simulink model "Model"  (R2021b)
settings: Solver=FixedStepAuto  StartTime=0.0  StopTime=T  FixedStep=0.1  RelTol=1e-3
values from neighbouring files (symbols this model uses):
  a = R_E + 550    [Model_script_291.m]
  A0 = eye(3)    [Model_script_291.m]
  actuators_matrix = [1 0 0; 0 1 0; 0 0 1]    [Model_script_291.m]
  alpha = deg2rad(11.5)    [Model_script_291.m]
  Area_mb = diag([A1 A2 A3 A4 A5 A6])    [Model_script_291.m]
  Area_sp = diag([A7 A8 A9 A10])    [Model_script_291.m]
  around_boresight = deg2rad(dms2degrees([0,0,around_boresight]))    [Model_script_291.m]
  cross_boresight = deg2rad(dms2degrees([0,0,cross_boresight]))    [Model_script_291.m]
  e = 0.0001824    [Model_script_291.m]
  epsilon = deg2rad(23.45)    [Model_script_291.m]
  H0 = ( g1_0^2 + g1_1^2 + h1_1^2 )^(1/2)    (= 3.0115258674e-05)    [Model_script_291.m]
  I = I_mb + I_depl    [Model_script_291.m]
  i = deg2rad(53.0545)    [Model_script_291.m]
  I_inv = inv(I)    [Model_script_291.m]
  i_matrix = [1 0 0; 0 cos(i) sin(i); 0 -sin(i) cos(i)]    [Model_script_291.m]
  Kb = 1e10    (= 10000000000)    [Model_script_291.m]
  Kd_slew = [5e-5; 5e-5; 5e-5]    [Model_script_291.m]
  Kd_tracking = [5e-3; 0.8*(5e-3); 5e-3]    [Model_script_291.m]
  Kp_slew = [5e-4; 5e-4; 5e-4]    [Model_script_291.m]
  Kp_tracking = [5e-2; 5e-2; 5e-2]    [Model_script_291.m]
  m = [0.01; 0.05; 0.01]    [Model_script_291.m]
  m_N_unit = zeros(size(m_N,1),size(m_N,2))    [Model_script_291.m]
  mu_E = astroConstants(13)    [Model_script_291.m]
  n = sqrt(mu_E/(a^3))    [Model_script_291.m]
  n4 = -n1    [Model_script_291.m]
  N_b_mb = [n1'; n2'; n3'; n4'; n5'; n6']    [Model_script_291.m]
  N_b_sp = [n7'; n8'; n9'; n10']    [Model_script_291.m]
  n_sun = 2*pi/T_sun    (= 1.99238499086e-07)    [Model_script_291.m]
  P = Fe/c    (= 4.52666666667e-06)    [Model_script_291.m]
  R_E = astroConstants(23)    [Model_script_291.m]
  r_mb = [base/2 0 0; 0 base/2 0; 0 0 height/2; -base/2 0 0; 0 -base/2 0; 0 0 -height/2]    [Model_script_291.m]
  r_sp = [0 length_p1/2+base/2 0; 0 length_p1/2+base/2 0; 0 -length_p2/2-base/2 0; 0 -length_p2/2-base/2 0]    [Model_script_291.m]
  rho_s_mb = 0.3    [Model_script_291.m]
  rho_s_sp = 0    [Model_script_291.m]
  Rs = astroConstants(2)    [Model_script_291.m]
  star_sensor_tolerance = deg2rad(star_sensor_tolerance)    [Model_script_291.m]
  theta0 = deg2rad(0)    [Model_script_291.m]
  unit = [1 0 0]'    [Model_script_291.m]
  v1 = [0 1 -1]'    [Model_script_291.m]
  v2 = [-1 0 1]'    [Model_script_291.m]
  v3 = [1 -1 0]'    [Model_script_291.m]
  w_0 = [wx_0 wy_0 wz_0]'    [Model_script_291.m]
  w_E = deg2rad(15.04)/3600    [Model_script_291.m]
  w_target = [0; 0; n]    [Model_script_291.m]
  weight = 1/6    (= 0.166666666667)    [Model_script_291.m]
  wy_0 = 0.7    [Model_script_291.m]
libraries: matrix_library x16, vrlib x12, dspmtrx3 x2, sharedutil x2
(part 1 of 2)
settings Model: Creator=sferl  LastModifiedBy=samuz

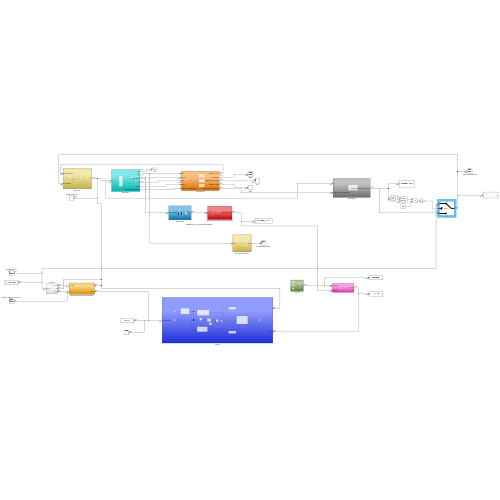
[thumbnail: Simulink's stored preview of the top-level diagram]
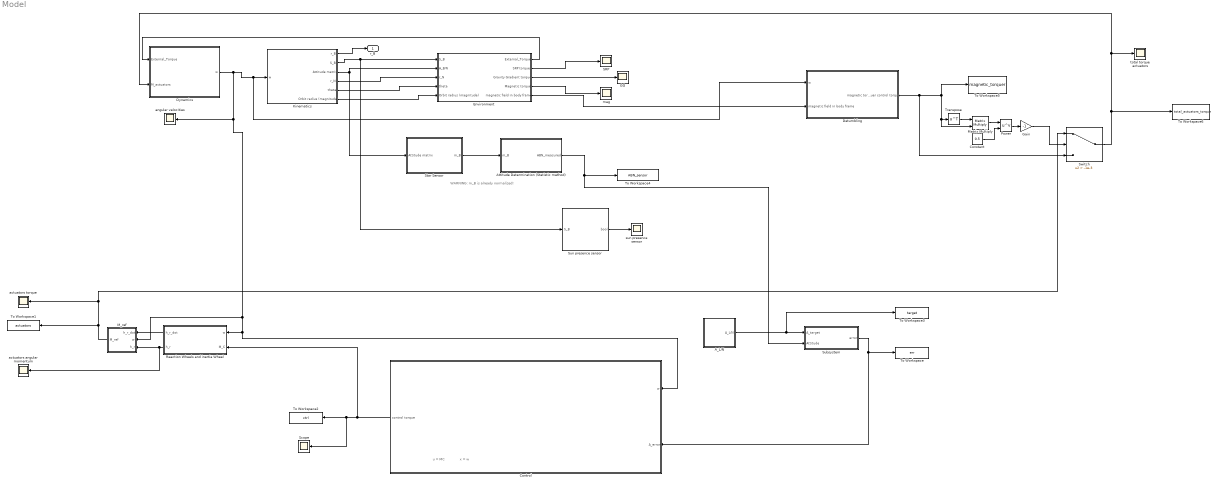
== system Model ==
  note: x = w
  note: u = MC
  note: WARNING: m_B is already normalized!
  A_L/N : Subsystem
  Attitude Determination (Statistic method) : Subsystem
  Constant : Constant  Value=0.5
  Control : Subsystem
  Detumbling : Subsystem
  Dynamics : Subsystem
  Environment : Subsystem
  GG : Scope
  Gain : Gain  Gain=-1
  Kinematics : Subsystem
  M_ref : Subsystem
  Matrix Multiply : Product  Multiplication=Matrix(*)
  Power : Math  Operator=pow  SaturateOnIntegerOverflow=on
  Reaction Wheels and inertia Wheel : Subsystem
  SRP : Scope
  Scope : Scope
  Star Sensor : Subsystem
  Subsystem : Subsystem
  Sun presence sensor : Subsystem
  Switch : Switch  Criteria=u2 > Threshold  Threshold=-1e-3
  To Workspace : ToWorkspace  VariableName=err  SampleTime=-1
  To Workspace1 : ToWorkspace  VariableName=actuators  SampleTime=-1
  To Workspace2 : ToWorkspace  VariableName=ctrl  SampleTime=-1
  To Workspace3 : ToWorkspace  VariableName=target  SampleTime=-1
  To Workspace4 : ToWorkspace  VariableName=ABN_sensor  SampleTime=-1
  To Workspace5 : ToWorkspace  VariableName=magnetic_torquer  SampleTime=-1
  To Workspace6 : ToWorkspace  VariableName=total_actuators_torque  SampleTime=-1
  Transpose : Math  Operator=transpose  SaturateOnIntegerOverflow=on
  actuators angular momentum : Scope
  actuators torque : Scope
  angular velocities : Scope
  mag : Scope
  sun presence sensor : Scope
  total torque actuators : Scope
  r_B : Outport
  wires:
  Kinematics/1(r_B) -> r_B/1
  Kinematics/3(Attitude matrix) -> Environment/2(A_B/N), Star Sensor/1(Attitude matrix)
  Star Sensor/1(m_B) -> Attitude Determination (Statistic method)/1(m_B)
  Kinematics/2(S_B) -> Sun presence sensor/1(S_B), Environment/1(S_B)
  Kinematics/4(r_N) -> Environment/3(r_N)
  Kinematics/5(theta) -> Environment/4(theta)
  Kinematics/6(Orbit radius (magnitude)) -> Environment/5(Orbit radius (magnitude))
  Environment/1(External_Torque) -> Dynamics/1(External_Torque)
  Attitude Determination (Statistic method)/1(ABN_measured) -> To Workspace4/1, Subsystem/2(Attitude)
  Subsystem/1(error) -> Control/2(A_error), To Workspace/1
  Environment/2(SRP torque) -> SRP/1
  Environment/3(Gravity Gradient torque) -> GG/1
  Environment/4(Magnetic torque) -> mag/1
  A_L/N/1(A_L/N) -> To Workspace3/1, Subsystem/1(A_target)
  Environment/5(magnetic field in body frame) -> Detumbling/2(magnetic field in body frame)
  Detumbling/1(magnetic torquer control torque) -> Switch/3, To Workspace5/1, Matrix Multiply/2, Transpose/1
  Dynamics/1(w) -> Detumbling/1(w), Kinematics/1(w), M_ref/2(w), Reaction Wheels and inertia Wheel/1(w), Control/1(w), angular velocities/1
  Transpose/1 -> Matrix Multiply/1
  Constant/1 -> Power/2
  Matrix Multiply/1 -> Power/1
  Power/1 -> Gain/1
  Gain/1 -> Switch/2
  Reaction Wheels and inertia Wheel/1(h_r_dot) -> M_ref/1(h_r_dot)
  Reaction Wheels and inertia Wheel/2(h_r) -> M_ref/3(h_r), actuators angular momentum/1
  Control/1(control torque) -> Reaction Wheels and inertia Wheel/2(M_C), Scope/1, To Workspace2/1
  M_ref/1(M_ref) -> To Workspace1/1, Switch/1, actuators torque/1
  Sun presence sensor/1(bool) -> sun presence sensor/1
  Switch/1 -> Dynamics/2(M_actuators), total torque actuators/1, To Workspace6/1

== system Model/A_L//N ==
  Matrix Concatenate : Concatenate  NumInputs=3  Mode=Multidimensional array  ConcatenateDimension=2
  first column of A_L/N : Subsystem
  second column of A_L/N : Subsystem
  third column of A_L/N : Subsystem
  A_L/N : Outport
  wires:
  second column of A_L/N/1(A_L/N (:,2)) -> Matrix Concatenate/2
  Matrix Concatenate/1 -> A_L/N/1
  first column of A_L/N/1(A_L/N (:,1)) -> Matrix Concatenate/1
  third column of A_L/N/1(A_L/N (:,3)) -> Matrix Concatenate/3

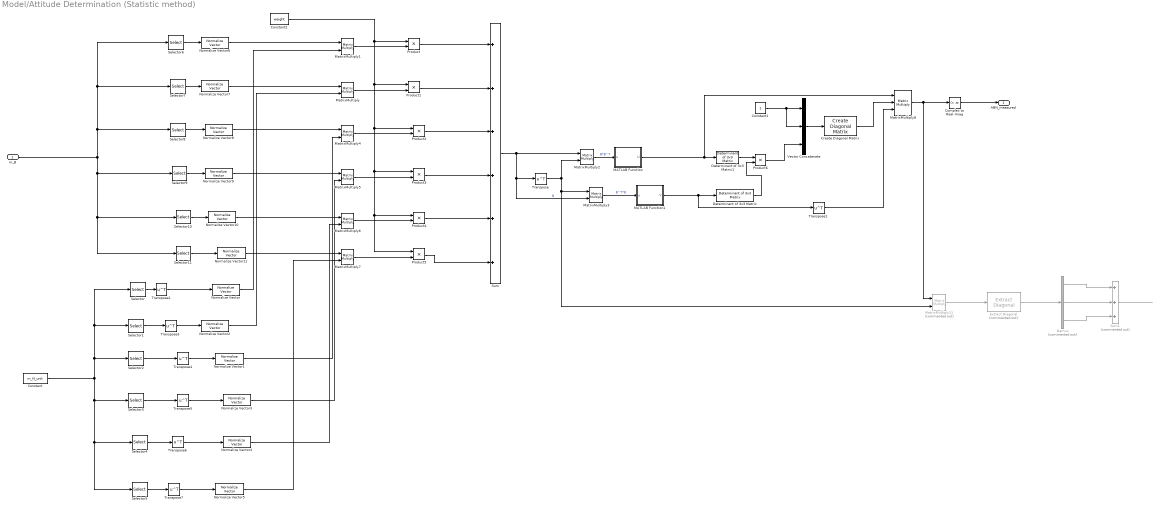
== system Model/Attitude Determination (Statistic method) ==
  m_B : Inport
  Complex to Real-Imag : ComplexToRealImag  Output=Real
  Constant : Constant  Value=m_N_unit
  Constant1 : Constant
  Constant2 : Constant  Value=weight
  Create Diagonal Matrix : dspmtrx3/Create Diagonal Matrix
      settings: SourceProductBaseCode=DS
  Demux : Demux  Commented=on  Outputs=3
  Determinant of 3x3 Matrix : sharedutil/Determinant of 3x3 Matrix  aMode=aMode
      settings: SourceProductBaseCode=AE,PW,DR,MT,UV,VE
  Determinant of 3x3 Matrix1 : sharedutil/Determinant of 3x3 Matrix  aMode=aMode
      settings: SourceProductBaseCode=AE,PW,DR,MT,UV,VE
  Extract Diagonal : dspmtrx3/Extract Diagonal  Commented=on
      settings: SourceProductBaseCode=DS
  MATLAB Function : MATLAB Function  TreatAsAtomicUnit=on
  MATLAB Function1 : MATLAB Function  TreatAsAtomicUnit=on
  MatrixMultiply{,1..7} (8 alike) : Product  Multiplication=Matrix(*)
  MatrixMultiply11 : Product  Commented=on  Multiplication=Matrix(*)
  MatrixMultiply8 : Product  Inputs=3  Multiplication=Matrix(*)
  Normalize Vector{,1..11} (12 alike) : vrlib/Utilities/Normalize Vector  maxzero=0
  Product{,1..6} (7 alike) : Product
  Selector : Selector  NumberOfDimensions=2  InputPortWidth=3  IndexOptions=Starting index (dialog),Starting index (dialog)  Indices=1,1  OutputSizes=3,1
  Selector1 : Selector  NumberOfDimensions=2  InputPortWidth=3  IndexOptions=Starting index (dialog),Starting index (dialog)  Indices=1,2  OutputSizes=3,1
  Selector10 : Selector  NumberOfDimensions=2  InputPortWidth=3  IndexOptions=Starting index (dialog),Starting index (dialog)  Indices=1,5  OutputSizes=3,1
  Selector11 : Selector  NumberOfDimensions=2  InputPortWidth=3  IndexOptions=Starting index (dialog),Starting index (dialog)  Indices=1,6  OutputSizes=3,1
  Selector2 : Selector  NumberOfDimensions=2  InputPortWidth=3  IndexOptions=Starting index (dialog),Starting index (dialog)  Indices=1,3  OutputSizes=3,1
  Selector3 : Selector  NumberOfDimensions=2  InputPortWidth=3  IndexOptions=Starting index (dialog),Starting index (dialog)  Indices=1,4  OutputSizes=3,1
  Selector4 : Selector  NumberOfDimensions=2  InputPortWidth=3  IndexOptions=Starting index (dialog),Starting index (dialog)  Indices=1,5  OutputSizes=3,1
  Selector5 : Selector  NumberOfDimensions=2  InputPortWidth=3  IndexOptions=Starting index (dialog),Starting index (dialog)  Indices=1,6  OutputSizes=3,1
  Selector6 : Selector  NumberOfDimensions=2  InputPortWidth=3  IndexOptions=Starting index (dialog),Starting index (dialog)  Indices=1,1  OutputSizes=3,1
  Selector7 : Selector  NumberOfDimensions=2  InputPortWidth=3  IndexOptions=Starting index (dialog),Starting index (dialog)  Indices=1,2  OutputSizes=3,1
  Selector8 : Selector  NumberOfDimensions=2  InputPortWidth=3  IndexOptions=Starting index (dialog),Starting index (dialog)  Indices=1,3  OutputSizes=3,1
  Selector9 : Selector  NumberOfDimensions=2  InputPortWidth=3  IndexOptions=Starting index (dialog),Starting index (dialog)  Indices=1,4  OutputSizes=3,1
  Sum : Sum  Inputs=++++++
  Sum1 : Sum  Commented=on  Inputs=+++
  Transpose{,1..7} (8 alike) : Math  Operator=transpose  SaturateOnIntegerOverflow=on
  Vector Concatenate : Concatenate  NumInputs=3
  ABN_measured : Outport
  wires:
  Transpose/1 -> MatrixMultiply11/2, MatrixMultiply3/1, MatrixMultiply2/2
  Constant2/1 -> Product3/1, Product4/1, Product5/1, Product2/1, Product1/1, Product/1
  Product2/1 -> Sum/3
  MatrixMultiply/1 -> Product1/2
  Product1/1 -> Sum/2
  MatrixMultiply7/1 -> Product5/2
  Sum/1 -> MatrixMultiply3/2, Transpose/1, MatrixMultiply2/1  "B"
  MatrixMultiply2/1 -> MATLAB Function/1(u)  "B*B^T"
  Product5/1 -> Sum/6
  MatrixMultiply5/1 -> Product3/2
  Product4/1 -> Sum/5
  Product/1 -> Sum/1
  MatrixMultiply4/1 -> Product2/2
  MatrixMultiply1/1 -> Product/2
  Product3/1 -> Sum/4
  MatrixMultiply6/1 -> Product4/2
  Selector1/1 -> Transpose3/1
  Selector3/1 -> Transpose5/1
  Selector4/1 -> Transpose6/1
  Selector2/1 -> Transpose4/1
  Selector5/1 -> Transpose7/1
  m_B/1 -> Selector6/1, Selector7/1, Selector8/1, Selector11/1, Selector10/1, Selector9/1
  Determinant of 3x3 Matrix1/1 -> Product6/1
  Determinant of 3x3 Matrix/1 -> Product6/2
  Constant1/1 -> Vector Concatenate/2, Vector Concatenate/1
  Product6/1 -> Vector Concatenate/3
  Vector Concatenate/1 -> Create Diagonal Matrix/1
  Create Diagonal Matrix/1 -> MatrixMultiply8/2
  MATLAB Function/1(U) -> MatrixMultiply8/1, Determinant of 3x3 Matrix1/1
  Transpose1/1 -> MatrixMultiply8/3
  MatrixMultiply8/1 -> Complex to Real-Imag/1, MatrixMultiply11/1
  MatrixMultiply3/1 -> MATLAB Function1/1(u)  "B^T*B"
  MATLAB Function1/1(V) -> Transpose1/1, Determinant of 3x3 Matrix/1
  MatrixMultiply11/1 -> Extract Diagonal/1
  Extract Diagonal/1 -> Demux/1
  Demux/1 -> Sum1/1
  Demux/2 -> Sum1/2
  Demux/3 -> Sum1/3
  Sum1/1 -> ?
  Selector6/1 -> Normalize Vector6/1
  Selector7/1 -> Normalize Vector7/1
  Selector8/1 -> Normalize Vector8/1
  Selector9/1 -> Normalize Vector9/1
  Selector10/1 -> Normalize Vector10/1
  Selector11/1 -> Normalize Vector11/1
  Selector/1 -> Transpose2/1
  Transpose3/1 -> Normalize Vector2/1
  Transpose2/1 -> Normalize Vector/1
  Transpose4/1 -> Normalize Vector1/1
  Transpose5/1 -> Normalize Vector3/1
  Transpose6/1 -> Normalize Vector4/1
  Transpose7/1 -> Normalize Vector5/1
  Normalize Vector/1 -> MatrixMultiply1/2
  Normalize Vector2/1 -> MatrixMultiply/2
  Normalize Vector1/1 -> MatrixMultiply4/2
  Normalize Vector3/1 -> MatrixMultiply5/2
  Normalize Vector4/1 -> MatrixMultiply6/2
  Normalize Vector5/1 -> MatrixMultiply7/2
  Normalize Vector6/1 -> MatrixMultiply1/1
  Normalize Vector7/1 -> MatrixMultiply/1
  Normalize Vector8/1 -> MatrixMultiply4/1
  Normalize Vector9/1 -> MatrixMultiply5/1
  Normalize Vector10/1 -> MatrixMultiply6/1
  Normalize Vector11/1 -> MatrixMultiply7/1
  Constant/1 -> Selector3/1, Selector4/1, Selector5/1, Selector/1, Selector1/1, Selector2/1
  Complex to Real-Imag/1 -> ABN_measured/1

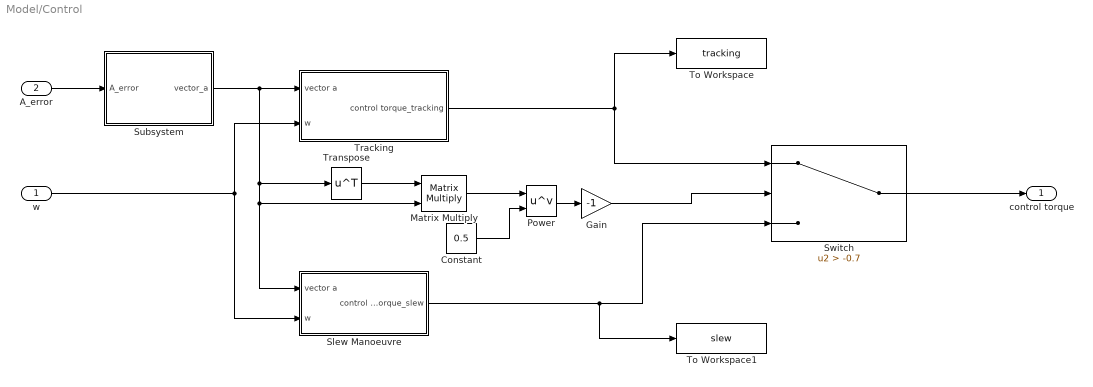
== system Model/Control ==
  w : Inport
  A_error : Inport  Port=2
  Constant : Constant  Value=0.5
  Gain : Gain  Gain=-1
  Matrix Multiply : Product  Multiplication=Matrix(*)
  Power : Math  Operator=pow  SaturateOnIntegerOverflow=on
  Slew Manoeuvre : Subsystem
  Subsystem : Subsystem
  Switch : Switch  Criteria=u2 > Threshold  Threshold=-0.7
  To Workspace : ToWorkspace  VariableName=tracking  SampleTime=-1
  To Workspace1 : ToWorkspace  VariableName=slew  SampleTime=-1
  Tracking : Subsystem
  Transpose : Math  Operator=transpose  SaturateOnIntegerOverflow=on
  control torque : Outport
  wires:
  w/1 -> Tracking/2(w), Slew Manoeuvre/2(w)
  Tracking/1(control torque_tracking) -> Switch/1, To Workspace/1
  A_error/1 -> Subsystem/1(A_error)
  Subsystem/1(vector_a) -> Slew Manoeuvre/1(vector a), Matrix Multiply/2, Transpose/1, Tracking/1(vector a)
  Slew Manoeuvre/1(control torque_slew) -> Switch/3, To Workspace1/1
  Switch/1 -> control torque/1
  Transpose/1 -> Matrix Multiply/1
  Matrix Multiply/1 -> Power/1
  Gain/1 -> Switch/2
  Constant/1 -> Power/2
  Power/1 -> Gain/1

== system Model/Detumbling ==
  w : Inport
  magnetic field in body frame : Inport  Port=2
  Mangetic Torquer : Subsystem
  magnetic torquer control torque : Outport
  wires:
  w/1 -> Mangetic Torquer/1(w)
  magnetic field in body frame/1 -> Mangetic Torquer/2(b)
  Mangetic Torquer/1(M_C) -> magnetic torquer control torque/1

== system Model/Dynamics ==
  External_Torque : Inport
  M_actuators : Inport  Port=2
  Constant : Constant  Value=I  VectorParams1D=off
  Constant1 : Constant  Value=I_inv  VectorParams1D=off
  Cross Product : matrix_library/Cross Product
      settings: SourceProductBaseCode=SL
  Integrator : Integrator  InitialCondition=w_0
  Product : Product  Multiplication=Matrix(*)
  Product1 : Product  Multiplication=Matrix(*)
  Sum : Sum  Inputs=|++
  Sum1 : Sum  Inputs=|++
  w : Outport
  wires:
  Product/1 -> Cross Product/1
  Constant/1 -> Product/1
  Constant1/1 -> Product1/1
  Integrator/1 -> Cross Product/2, Product/2, w/1  "w"
  Product1/1 -> Integrator/1  "w_dot"
  Cross Product/1 -> Sum/2
  Sum/1 -> Product1/2
  External_Torque/1 -> Sum1/1
  M_actuators/1 -> Sum1/2
  Sum1/1 -> Sum/1

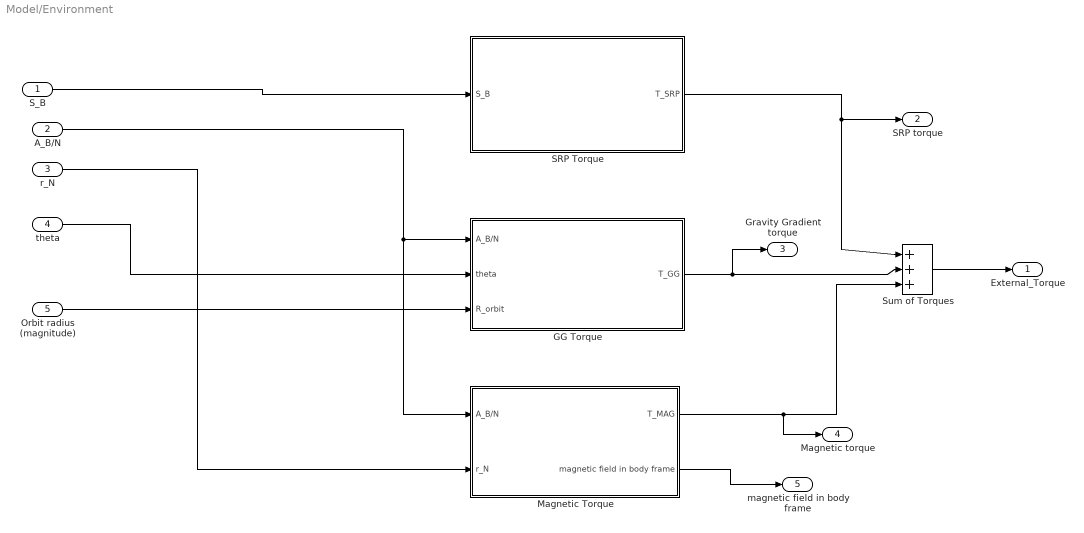
== system Model/Environment ==
  S_B : Inport
  A_B/N : Inport  Port=2
  r_N : Inport  Port=3
  theta : Inport  Port=4
  Orbit radius (magnitude) : Inport  Port=5
  GG Torque : Subsystem
  Magnetic Torque : Subsystem
  SRP Torque : Subsystem
  Sum of Torques : Sum  Inputs=+|+|+  CollapseMode=Specified dimension
  External_Torque : Outport
  SRP torque : Outport  Port=2
  Gravity Gradient torque : Outport  Port=3
  Magnetic torque : Outport  Port=4
  magnetic field in body frame : Outport  Port=5
  wires:
  SRP Torque/1(T_SRP) -> SRP torque/1, Sum of Torques/1
  r_N/1 -> Magnetic Torque/2(r_N)
  GG Torque/1(T_GG) -> Gravity Gradient torque/1, Sum of Torques/2
  A_B/N/1 -> Magnetic Torque/1(A_B/N), GG Torque/1(A_B/N)
  Orbit radius (magnitude)/1 -> GG Torque/3(R_orbit)
  Magnetic Torque/1(T_MAG) -> Magnetic torque/1, Sum of Torques/3
  Sum of Torques/1 -> External_Torque/1
  S_B/1 -> SRP Torque/1(S_B)
  theta/1 -> GG Torque/2(theta)
  Magnetic Torque/2(magnetic field in body frame) -> magnetic field in body frame/1

== system Model/Kinematics ==
  w : Inport
  Sun direction with respect to body frame (already normalized!) : Subsystem
  "radius of orbit in body frame and transformation matrix from inertial frame to body frame " : Subsystem
  r_B : Outport
  S_B : Outport  Port=2
  Attitude matrix : Outport  Port=3
  r_N : Outport  Port=4
  theta : Outport  Port=5
  Orbit radius (magnitude) : Outport  Port=6
  wires:
  "radius of orbit in body frame and transformation matrix from inertial frame to body frame "/1(r_B) -> r_B/1
  w/1 -> "radius of orbit in body frame and transformation matrix from inertial frame to body frame "/1(w)
  Sun direction with respect to body frame (already normalized!)/1(S_B) -> S_B/1
  "radius of orbit in body frame and transformation matrix from inertial frame to body frame "/3(r_N) -> r_N/1
  "radius of orbit in body frame and transformation matrix from inertial frame to body frame "/4(theta) -> theta/1
  "radius of orbit in body frame and transformation matrix from inertial frame to body frame "/5(R_orbit) -> Orbit radius (magnitude)/1
  "radius of orbit in body frame and transformation matrix from inertial frame to body frame "/2(A_B/N) -> Attitude matrix/1, Sun direction with respect to body frame (already normalized!)/1(A_B/N)

== system Model/M_ref ==
  h_r_dot : Inport
  w : Inport  Port=2
  h_r : Inport  Port=3
  Constant : Constant  Value=actuators_matrix
  Constant1 : Constant  Value=actuators_matrix
  Cross Product : matrix_library/Cross Product
      settings: SourceProductBaseCode=SL
  Gain : Gain  Gain=-1
  MatrixMultiply : Product  Multiplication=Matrix(*)
  MatrixMultiply1 : Product  Multiplication=Matrix(*)
  Sum : Sum  Inputs=|++
  M_ref : Outport
  wires:
  MatrixMultiply1/1 -> Cross Product/2
  MatrixMultiply/1 -> Sum/1
  Sum/1 -> Gain/1
  Constant/1 -> MatrixMultiply/1
  h_r_dot/1 -> MatrixMultiply/2
  Cross Product/1 -> Sum/2
  Gain/1 -> M_ref/1
  w/1 -> Cross Product/1
  Constant1/1 -> MatrixMultiply1/1
  h_r/1 -> MatrixMultiply1/2

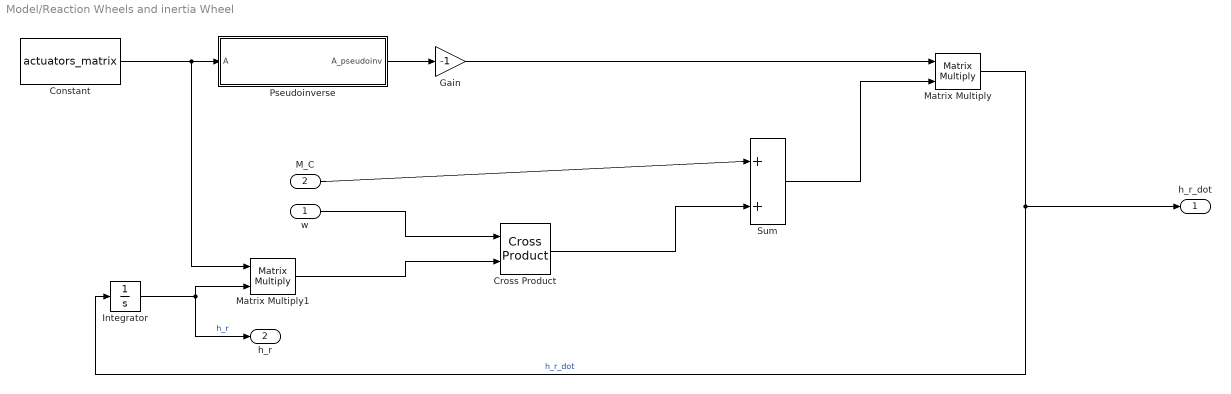
== system Model/Reaction Wheels and inertia Wheel ==
  w : Inport
  M_C : Inport  Port=2
  Constant : Constant  Value=actuators_matrix
  Cross Product : matrix_library/Cross Product
      settings: SourceProductBaseCode=SL
  Gain : Gain  Gain=-1
  Integrator : Integrator  InitialCondition=[0; wy_0; 0]
  Matrix Multiply : Product  Multiplication=Matrix(*)
  Matrix Multiply1 : Product  Multiplication=Matrix(*)
  Pseudoinverse : MATLAB Function  TreatAsAtomicUnit=on
  Sum : Sum  Inputs=|++
  h_r_dot : Outport
  h_r : Outport  Port=2
  wires:
  Constant/1 -> Matrix Multiply1/1, Pseudoinverse/1(A)
  Pseudoinverse/1(A_pseudoinv) -> Gain/1
  Gain/1 -> Matrix Multiply/1
  M_C/1 -> Sum/1
  w/1 -> Cross Product/1
  Matrix Multiply/1 -> h_r_dot/1, Integrator/1  "h_r_dot"
  Integrator/1 -> h_r/1, Matrix Multiply1/2  "h_r"
  Matrix Multiply1/1 -> Cross Product/2
  Cross Product/1 -> Sum/2
  Sum/1 -> Matrix Multiply/2

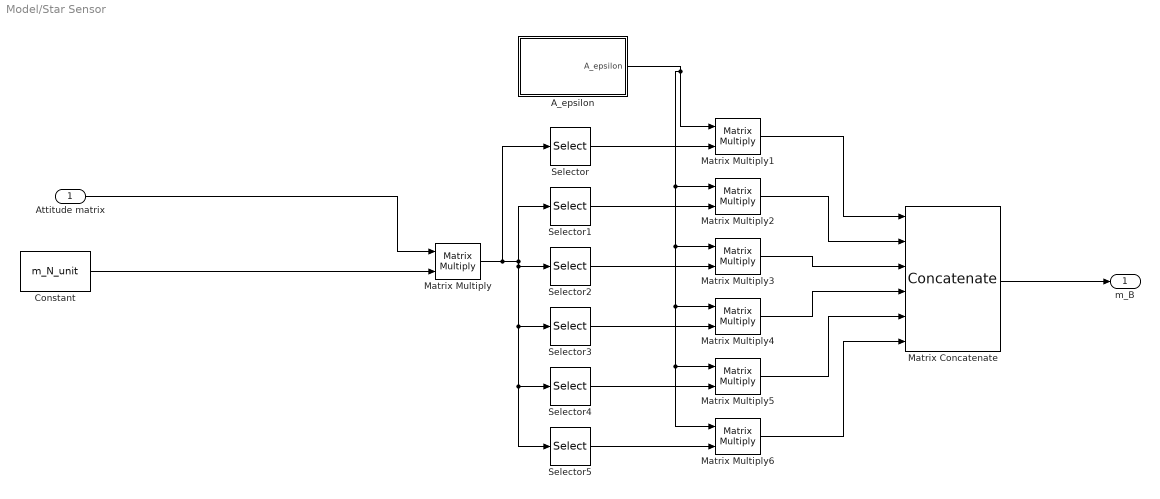
== system Model/Star Sensor ==
  Attitude matrix : Inport
  A_epsilon : Subsystem
  Constant : Constant  Value=m_N_unit
  Matrix Concatenate : Concatenate  NumInputs=6  Mode=Multidimensional array  ConcatenateDimension=2
  Matrix Multiply{,1..6} (7 alike) : Product  Multiplication=Matrix(*)
  Selector : Selector  NumberOfDimensions=2  InputPortWidth=3  IndexOptions=Starting index (dialog),Starting index (dialog)  Indices=1,1  OutputSizes=3,1
  Selector1 : Selector  NumberOfDimensions=2  InputPortWidth=3  IndexOptions=Starting index (dialog),Starting index (dialog)  Indices=1,2  OutputSizes=3,1
  Selector2 : Selector  NumberOfDimensions=2  InputPortWidth=3  IndexOptions=Starting index (dialog),Starting index (dialog)  Indices=1,3  OutputSizes=3,1
  Selector3 : Selector  NumberOfDimensions=2  InputPortWidth=3  IndexOptions=Starting index (dialog),Starting index (dialog)  Indices=1,4  OutputSizes=3,1
  Selector4 : Selector  NumberOfDimensions=2  InputPortWidth=3  IndexOptions=Starting index (dialog),Starting index (dialog)  Indices=1,5  OutputSizes=3,1
  Selector5 : Selector  NumberOfDimensions=2  InputPortWidth=3  IndexOptions=Starting index (dialog),Starting index (dialog)  Indices=1,6  OutputSizes=3,1
  m_B : Outport
  wires:
  Attitude matrix/1 -> Matrix Multiply/1
  Constant/1 -> Matrix Multiply/2
  Matrix Multiply/1 -> Selector5/1, Selector4/1, Selector3/1, Selector2/1, Selector1/1, Selector/1
  A_epsilon/1(A_epsilon) -> Matrix Multiply6/1, Matrix Multiply5/1, Matrix Multiply4/1, Matrix Multiply3/1, Matrix Multiply2/1, Matrix Multiply1/1
  Selector/1 -> Matrix Multiply1/2
  Selector1/1 -> Matrix Multiply2/2
  Selector2/1 -> Matrix Multiply3/2
  Selector3/1 -> Matrix Multiply4/2
  Selector4/1 -> Matrix Multiply5/2
  Selector5/1 -> Matrix Multiply6/2
  Matrix Multiply1/1 -> Matrix Concatenate/1
  Matrix Multiply2/1 -> Matrix Concatenate/2
  Matrix Multiply3/1 -> Matrix Concatenate/3
  Matrix Multiply4/1 -> Matrix Concatenate/4
  Matrix Multiply5/1 -> Matrix Concatenate/5
  Matrix Multiply6/1 -> Matrix Concatenate/6
  Matrix Concatenate/1 -> m_B/1

== system Model/Subsystem ==
  note: A measured
  note: A target
  A_target : Inport
  Attitude : Inport  Port=2
  Matrix Multiply : Product  Multiplication=Matrix(*)
  Transpose : Math  Operator=transpose  SaturateOnIntegerOverflow=on
  error : Outport
  wires:
  Transpose/1 -> Matrix Multiply/2
  Matrix Multiply/1 -> error/1
  Attitude/1 -> Matrix Multiply/1
  A_target/1 -> Transpose/1

== system Model/Sun presence sensor ==
  note: sun presence sensor gives me a boolean output to understand if star sensor points the Sun or not along the orbit
  note: if bool = 0 then sun sensor is turned off at least once
  note: If cos(angle) is negative then the star sensor is not pointing towards the Sun -> star sensor is turned on and I compute the attitude with its measurements (see attitude determination block)
  note: if cos(angle) is positive then the star sensor is pointing towards the Sun -> star sensor must be turned off and I activate the observer to estimate the attitude from the latest given measurements
  S_B : Inport
  Constant : Constant  Value=n4
  Constant1 : Constant  Value=0
  Constant2 : Constant
  Constant3 : Constant  Value=star_sensor_tolerance
  Cos : Trigonometry  Operator=cos
  Dot Product : DotProduct  InputSameDT=on  OutDataTypeStr=Inherit: Inherit via internal rule
  Sum : Sum  Inputs=+-
  Switch : Switch  Criteria=u2 > Threshold
  bool : Outport
  wires:
  S_B/1 -> Dot Product/1
  Dot Product/1 -> Sum/1  "cos(angle_between_n4_and_Sb)"
  Constant1/1 -> Switch/1  "star sensor points Sun"
  Constant2/1 -> Switch/3  "star sensor doesn't point Sun"
  Constant3/1 -> Cos/1
  Cos/1 -> Sum/2
  Sum/1 -> Switch/2
  Constant/1 -> Dot Product/2
  Switch/1 -> bool/1

== system Model/A_L//N/first column of A_L//N ==
  Constant : Constant  Value=0
  Cos : Trigonometry  Operator=cos
  Gain : Gain  Gain=-1
  Sin : Trigonometry
  Vector Concatenate : Concatenate  NumInputs=3
  argument of periodic functions : Subsystem
  argument of periodic functions1 : Subsystem
  A_L/N (:,1) : Outport
  wires:
  argument of periodic functions/1(n*t) -> Cos/1
  Constant/1 -> Vector Concatenate/3
  Cos/1 -> Vector Concatenate/1
  Vector Concatenate/1 -> A_L/N (:,1)/1
  Gain/1 -> Vector Concatenate/2
  Sin/1 -> Gain/1
  argument of periodic functions1/1(n*t) -> Sin/1

== system Model/A_L//N/second column of A_L//N ==
  Constant : Constant  Value=0
  Cos : Trigonometry
  Sin : Trigonometry  Operator=cos
  Vector Concatenate : Concatenate  NumInputs=3
  argument of periodic functions : Subsystem
  argument of periodic functions1 : Subsystem
  A_L/N (:,2) : Outport
  wires:
  argument of periodic functions/1(n*t) -> Cos/1
  Constant/1 -> Vector Concatenate/3
  Cos/1 -> Vector Concatenate/1
  Vector Concatenate/1 -> A_L/N (:,2)/1
  Sin/1 -> Vector Concatenate/2
  argument of periodic functions1/1(n*t) -> Sin/1

== system Model/A_L//N/third column of A_L//N ==
  Constant : Constant
  Constant1 : Constant  Value=0
  Constant2 : Constant  Value=0
  Vector Concatenate : Concatenate  NumInputs=3
  A_L/N (:,3) : Outport
  wires:
  Constant/1 -> Vector Concatenate/3
  Vector Concatenate/1 -> A_L/N (:,3)/1
  Constant1/1 -> Vector Concatenate/2
  Constant2/1 -> Vector Concatenate/1

== system Model/Control/Slew Manoeuvre ==
  vector a : Inport
  w : Inport  Port=2
  Constant5 : Constant  Value=Kp_slew
  Constant8 : Constant  Value=Kd_slew
  Matrix Multiply : Product
  Matrix Multiply1 : Product
  Sum : Sum  Inputs=|++
  control torque_slew : Outport
  wires:
  w/1 -> Matrix Multiply1/2
  Sum/1 -> control torque_slew/1
  Matrix Multiply1/1 -> Sum/2
  Matrix Multiply/1 -> Sum/1
  Constant8/1 -> Matrix Multiply1/1
  Constant5/1 -> Matrix Multiply/1
  vector a/1 -> Matrix Multiply/2

== system Model/Control/Subsystem ==
  A_error : Inport
  -az : Selector  NumberOfDimensions=2  InputPortWidth=3  IndexOptions=Starting index (dialog),Starting index (dialog)  Indices=2,1  OutputSizes=1,1
  Gain : Gain  Gain=-1
  ax : Selector  NumberOfDimensions=2  InputPortWidth=3  IndexOptions=Starting index (dialog),Starting index (dialog)  Indices=2,3  OutputSizes=1,1
  ay : Selector  NumberOfDimensions=2  InputPortWidth=3  IndexOptions=Starting index (dialog),Starting index (dialog)  Indices=3,1  OutputSizes=1,1
  vector a : Mux  Inputs=3
  vector_a : Outport
  wires:
  A_error/1 -> ax/1, ay/1, -az/1
  ay/1 -> vector a/2
  ax/1 -> vector a/1
  Gain/1 -> vector a/3
  -az/1 -> Gain/1
  vector a/1 -> vector_a/1

== system Model/Control/Tracking ==
  vector a : Inport
  w : Inport  Port=2
  Constant5 : Constant  Value=Kp_tracking
  Constant8 : Constant  Value=Kd_tracking
  Constant9 : Constant  Value=w_target
  Matrix Multiply : Product
  Matrix Multiply1 : Product
  Sum : Sum  Inputs=|++
  Sum1 : Sum  Inputs=+-
  control torque_tracking : Outport
  wires:
  Sum1/1 -> Matrix Multiply1/2
  Sum/1 -> control torque_tracking/1
  w/1 -> Sum1/1
  Constant9/1 -> Sum1/2
  Matrix Multiply1/1 -> Sum/2
  Matrix Multiply/1 -> Sum/1
  Constant8/1 -> Matrix Multiply1/1
  Constant5/1 -> Matrix Multiply/1
  vector a/1 -> Matrix Multiply/2

== system Model/Detumbling/Mangetic Torquer ==
  note: B_dot
  w : Inport
  b : Inport  Port=2
  Constant : Constant  Value=Kb
  Cross Product : matrix_library/Cross Product
      settings: SourceProductBaseCode=SL
  Demux : Demux  Outputs=3
  Gain : Gain  Gain=-1
  Gain1 : Gain  Gain=-1
  Matrix Multiply : Product  Multiplication=Matrix(*)
  Matrix Multiply1 : Product
  w_hat : Subsystem
  M_C : Outport
  wires:
  Matrix Multiply/1 -> Matrix Multiply1/2
  Constant/1 -> Gain/1
  b/1 -> Cross Product/2, Matrix Multiply/2
  Gain/1 -> Matrix Multiply1/1
  Gain1/1 -> Matrix Multiply/1
  Demux/3 -> w_hat/3(w_z)  "w_z"
  Matrix Multiply1/1 -> Cross Product/1
  Demux/1 -> w_hat/1(w_x)  "w_x"
  Demux/2 -> w_hat/2(w_y)  "w_y"
  w_hat/1(w_hat) -> Gain1/1
  Cross Product/1 -> M_C/1
  w/1 -> Demux/1

== system Model/Environment/GG Torque ==
  A_B/N : Inport
  theta : Inport  Port=2
  R_orbit : Inport  Port=3
  Gravity Gradient : Subsystem
  Transformation from A_B/N to A_B/L : Subsystem
  T_GG : Outport
  wires:
  Gravity Gradient/1(T_GG) -> T_GG/1
  Transformation from A_B/N to A_B/L/1(A_B/L) -> Gravity Gradient/1(A_BL)
  A_B/N/1 -> Transformation from A_B/N to A_B/L/1(A_B/N)
  theta/1 -> Transformation from A_B/N to A_B/L/2(theta)
  R_orbit/1 -> Gravity Gradient/2(R_orbit)

== system Model/Environment/Magnetic Torque ==
  A_B/N : Inport
  r_N : Inport  Port=2
  Cross Product : matrix_library/Cross Product
      settings: SourceProductBaseCode=SL
  magnetic field of Earth (modelled as dipole) in body frame : Subsystem
  parasitic magnetic torque : Constant  Value=m
  T_MAG : Outport
  magnetic field in body frame : Outport  Port=2
  wires:
  A_B/N/1 -> magnetic field of Earth (modelled as dipole) in body frame/1(A_B/N)
  magnetic field of Earth (modelled as dipole) in body frame/1(b_B) -> magnetic field in body frame/1, Cross Product/2
  parasitic magnetic torque/1 -> Cross Product/1
  Cross Product/1 -> T_MAG/1
  r_N/1 -> magnetic field of Earth (modelled as dipole) in body frame/2(r_N)

== system Model/Environment/SRP Torque ==
  S_B : Inport
  Matrix Concatenate : Concatenate  Mode=Multidimensional array
  SRP Force on spacecraft main body : Subsystem
  SRP Force on spacecraft solar panels : Subsystem
  SRP Torque on spacecraft main body : Subsystem
  SRP Torque on spacecraft solar panels : Subsystem
  Sum of Elements : Sum  Inputs=+  CollapseMode=Specified dimension
  Transpose : Math  Operator=transpose  SaturateOnIntegerOverflow=on
  T_SRP : Outport
  wires:
  S_B/1 -> SRP Force on spacecraft main body/1(S_B), SRP Force on spacecraft solar panels/1(S_B)
  SRP Force on spacecraft solar panels/1(F_sp) -> SRP Torque on spacecraft solar panels/1(F_sp)
  SRP Force on spacecraft main body/1(F_mb) -> SRP Torque on spacecraft main body/1(F_mb)
  SRP Torque on spacecraft solar panels/1(T_sp) -> Matrix Concatenate/2
  SRP Torque on spacecraft main body/1(T_mb) -> Matrix Concatenate/1
  Sum of Elements/1 -> Transpose/1
  Transpose/1 -> T_SRP/1
  Matrix Concatenate/1 -> Sum of Elements/1

== system Model/Kinematics/Sun direction with respect to body frame (already normalized!) ==
  note: I divide the vector for its magnitude (Rs): this is the normalization!
  A_B/N : Inport
  Constant7 : Constant  Value=1/Rs
  MatrixMultiply : Product  Multiplication=Matrix(*)
  Product5 : Product
  S_N : Subsystem
  S_B : Outport
  wires:
  S_N/1(Out1) -> MatrixMultiply/2
  A_B/N/1 -> MatrixMultiply/1
  Constant7/1 -> Product5/1
  MatrixMultiply/1 -> Product5/2
  Product5/1 -> S_B/1

== system Model/Kinematics/radius of orbit in body frame and transformation matrix from inertial frame to body frame  ==
  w : Inport
  MatrixMultiply1 : Product  Multiplication=Matrix(*)
  finder of A_B/N(t) : Subsystem
  orthonormalization of matrix A(t) : Subsystem
  radius of orbit in the inertial reference frame : Subsystem
  r_B : Outport
  A_B/N : Outport  Port=2
  r_N : Outport  Port=3
  theta : Outport  Port=4
  R_orbit : Outport  Port=5
  wires:
  finder of A_B/N(t)/1(A(t)) -> orthonormalization of matrix A(t)/1(A(t))
  orthonormalization of matrix A(t)/1(A_orthonorm) -> A_B/N/1, MatrixMultiply1/2
  MatrixMultiply1/1 -> r_B/1
  radius of orbit in the inertial reference frame/2(r_N) -> MatrixMultiply1/1, r_N/1
  w/1 -> finder of A_B/N(t)/1(w)
  radius of orbit in the inertial reference frame/1(theta) -> theta/1
  radius of orbit in the inertial reference frame/3(R_orbit) -> R_orbit/1

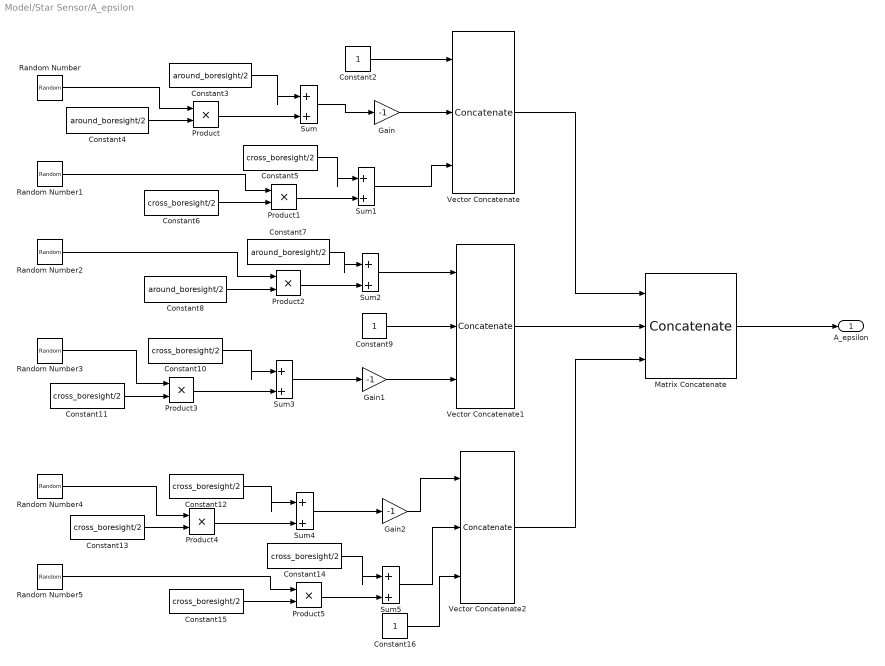
== system Model/Star Sensor/A_epsilon ==
  Constant{5..6,10..15} (8 alike) : Constant  Value=cross_boresight/2
  Constant16 : Constant
  Constant2 : Constant
  Constant{3..4,7..8} (4 alike) : Constant  Value=around_boresight/2
  Constant9 : Constant
  Gain : Gain  Gain=-1
  Gain1 : Gain  Gain=-1
  Gain2 : Gain  Gain=-1
  Matrix Concatenate : Concatenate  NumInputs=3  Mode=Multidimensional array  ConcatenateDimension=2
  Product{,1..5} (6 alike) : Product
  Random Number{,1..5} (6 alike) : RandomNumber  Variance=0.16  SampleTime=0.1
  Sum{,1..5} (6 alike) : Sum  Inputs=|++
  Vector Concatenate : Concatenate  NumInputs=3  Mode=Multidimensional array
  Vector Concatenate1 : Concatenate  NumInputs=3  Mode=Multidimensional array
  Vector Concatenate2 : Concatenate  NumInputs=3  Mode=Multidimensional array
  A_epsilon : Outport
  wires:
  Constant10/1 -> Sum3/1
  Random Number/1 -> Product/1
  Constant12/1 -> Sum4/1
  Vector Concatenate2/1 -> Matrix Concatenate/3
  Constant11/1 -> Product3/2
  Sum/1 -> Gain/1
  Vector Concatenate1/1 -> Matrix Concatenate/2
  Constant3/1 -> Sum/1
  Product1/1 -> Sum1/2
  Constant15/1 -> Product5/2
  Constant16/1 -> Vector Concatenate2/3
  Product5/1 -> Sum5/2
  Constant13/1 -> Product4/2
  Product3/1 -> Sum3/2
  Constant6/1 -> Product1/2
  Product2/1 -> Sum2/2
  Constant7/1 -> Sum2/1
  Constant4/1 -> Product/2
  Constant9/1 -> Vector Concatenate1/2
  Constant8/1 -> Product2/2
  Sum2/1 -> Vector Concatenate1/1
  Gain/1 -> Vector Concatenate/2
  Sum3/1 -> Gain1/1
  Product4/1 -> Sum4/2
  Constant2/1 -> Vector Concatenate/1
  Sum5/1 -> Vector Concatenate2/2
  Vector Concatenate/1 -> Matrix Concatenate/1
  Product/1 -> Sum/2
  Sum1/1 -> Vector Concatenate/3
  Constant14/1 -> Sum5/1
  Gain1/1 -> Vector Concatenate1/3
  Gain2/1 -> Vector Concatenate2/1
  Constant5/1 -> Sum1/1
  Sum4/1 -> Gain2/1
  Matrix Concatenate/1 -> A_epsilon/1
  Random Number1/1 -> Product1/1
  Random Number2/1 -> Product2/1
  Random Number3/1 -> Product3/1
  Random Number4/1 -> Product4/1
  Random Number5/1 -> Product5/1

== system Model/A_L//N/first column of A_L//N/argument of periodic functions ==
  Clock : Clock
  Constant : Constant  Value=n
  Dot Product : DotProduct  InputSameDT=on  OutDataTypeStr=Inherit: Inherit via internal rule
  n*t : Outport
  wires:
  Clock/1 -> Dot Product/1
  Dot Product/1 -> n*t/1
  Constant/1 -> Dot Product/2

== system Model/A_L//N/first column of A_L//N/argument of periodic functions1 ==
  Clock : Clock
  Constant : Constant  Value=n
  Dot Product : DotProduct  InputSameDT=on  OutDataTypeStr=Inherit: Inherit via internal rule
  n*t : Outport
  wires:
  Clock/1 -> Dot Product/1
  Dot Product/1 -> n*t/1
  Constant/1 -> Dot Product/2

== system Model/A_L//N/second column of A_L//N/argument of periodic functions ==
  Clock : Clock
  Constant : Constant  Value=n
  Dot Product : DotProduct  InputSameDT=on  OutDataTypeStr=Inherit: Inherit via internal rule
  n*t : Outport
  wires:
  Clock/1 -> Dot Product/1
  Dot Product/1 -> n*t/1
  Constant/1 -> Dot Product/2

== system Model/A_L//N/second column of A_L//N/argument of periodic functions1 ==
  Clock : Clock
  Constant : Constant  Value=n
  Dot Product : DotProduct  InputSameDT=on  OutDataTypeStr=Inherit: Inherit via internal rule
  n*t : Outport
  wires:
  Clock/1 -> Dot Product/1
  Dot Product/1 -> n*t/1
  Constant/1 -> Dot Product/2

== system Model/Detumbling/Mangetic Torquer/w_hat ==
  w_x : Inport
  w_y : Inport  Port=2
  w_z : Inport  Port=3
  Matrix Concatenate : Concatenate  NumInputs=3  Mode=Multidimensional array  ConcatenateDimension=2
  Scope : Scope  NumInputPorts=3
  Subsystem : Subsystem
  Subsystem1 : Subsystem
  Subsystem2 : Subsystem
  w_hat : Outport
  wires:
  w_y/1 -> Subsystem1/2(w_y), Subsystem/2(w_y), Subsystem2/2(w_y), Scope/2
  w_z/1 -> Subsystem2/3(w_z), Subsystem/3(w_z), Subsystem1/3(w_z), Scope/3
  w_x/1 -> Subsystem2/1(w_x), Subsystem/1(w_x), Subsystem1/1(w_x), Scope/1
  Subsystem2/1(Out1) -> Matrix Concatenate/3
  Subsystem1/1(Out1) -> Matrix Concatenate/2
  Subsystem/1(Out1) -> Matrix Concatenate/1
  Matrix Concatenate/1 -> w_hat/1

== system Model/Environment/GG Torque/Gravity Gradient ==
  A_BL : Inport
  R_orbit : Inport  Port=2
  Constant4 : Constant  Value=I
  Cross Product1 : matrix_library/Cross Product
      settings: SourceProductBaseCode=SL
  MatrixMultiply4 : Product  Multiplication=Matrix(*)
  Product : Product
  To Workspace : ToWorkspace  VariableName=c_vector  SampleTime=-1
  creation of coefficient 3*mu_E/(R^3) : Subsystem
  creation of vector c : Subsystem
  T_GG : Outport
  wires:
  Constant4/1 -> MatrixMultiply4/1
  MatrixMultiply4/1 -> Cross Product1/2
  Cross Product1/1 -> Product/2
  Product/1 -> T_GG/1
  creation of vector c/1(c) -> To Workspace/1, MatrixMultiply4/2, Cross Product1/1
  A_BL/1 -> creation of vector c/1(A_BL)
  R_orbit/1 -> creation of coefficient 3*mu_E/(R^3)/1(In1)
  creation of coefficient 3*mu_E/(R^3)/1(Out1) -> Product/1

== system Model/Environment/GG Torque/Transformation from A_B//N to A_B//L ==
  A_B/N : Inport
  theta : Inport  Port=2
  Constant : Constant  Value=i_matrix
  Matrix Multiply : Product  Multiplication=Matrix(*)
  MatrixMultiply1 : Product  Multiplication=Matrix(*)
  Transpose : Math  Operator=transpose  SaturateOnIntegerOverflow=on
  creation of A L/N : Subsystem
  A_B/L : Outport
  wires:
  A_B/N/1 -> MatrixMultiply1/1
  Transpose/1 -> MatrixMultiply1/2
  MatrixMultiply1/1 -> A_B/L/1  "A_BL"
  creation of A L/N/1(A_L/N) -> Matrix Multiply/1
  Constant/1 -> Matrix Multiply/2
  Matrix Multiply/1 -> Transpose/1
  theta/1 -> creation of A L/N/1(theta)

== system Model/Environment/Magnetic Torque/magnetic field of Earth (modelled as dipole) in body frame ==
  A_B/N : Inport
  r_N : Inport  Port=2
  Matrix Multiply : Product  Multiplication=Matrix(*)
  b_N : Subsystem
  b_B : Outport
  wires:
  b_N/1(b_N) -> Matrix Multiply/2
  r_N/1 -> b_N/1(r_N)
  A_B/N/1 -> Matrix Multiply/1
  Matrix Multiply/1 -> b_B/1

== system Model/Environment/SRP Torque/SRP Force on spacecraft main body ==
  S_B : Inport
  (1-rho_s)*Sb : Subsystem
  (2*rho_s*cos(theta)+2/3*rho_d)*Nb : Subsystem
  -PA*cos(theta) : Subsystem
  MatrixMultiply3 : Product  Multiplication=Matrix(*)
  Sum2 : Sum  Inputs=|++
  Switch to compute only force of exposed surfaces : Subsystem  TreatAsAtomicUnit=on
  compiute angle between incoming radiation and surface : Subsystem
  F_mb : Outport
  wires:
  S_B/1 -> (1-rho_s)*Sb/1(In1), compiute angle between incoming radiation and surface/1(S_B)
  compiute angle between incoming radiation and surface/1(cos_theta_mb) -> Switch to compute only force of exposed surfaces/1(In1)
  -PA*cos(theta)/1(Out1) -> MatrixMultiply3/1
  Sum2/1 -> MatrixMultiply3/2
  (1-rho_s)*Sb/1(Out1) -> Sum2/1
  (2*rho_s*cos(theta)+2/3*rho_d)*Nb/1(Out1) -> Sum2/2
  MatrixMultiply3/1 -> F_mb/1
  Switch to compute only force of exposed surfaces/1(Out1) -> -PA*cos(theta)/1(Input), (2*rho_s*cos(theta)+2/3*rho_d)*Nb/1(In1)

== system Model/Environment/SRP Torque/SRP Force on spacecraft solar panels ==
  S_B : Inport
  (1-rho_s)*Sb : Subsystem
  (2*rho_s*cos(theta)+2/3*rho_d)*Nb : Subsystem
  -PA*cos(theta) : Subsystem
  MatrixMultiply3 : Product  Multiplication=Matrix(*)
  Sum2 : Sum  Inputs=|++
  Switch to compute only force of exposed surfaces : Subsystem  TreatAsAtomicUnit=on
  compiute angle between incoming radiation and surface : Subsystem
  F_sp : Outport
  wires:
  S_B/1 -> (1-rho_s)*Sb/1(In1), compiute angle between incoming radiation and surface/1(S_B)
  compiute angle between incoming radiation and surface/1(cos_theta_sp) -> Switch to compute only force of exposed surfaces/1(In1)
  -PA*cos(theta)/1(Out1) -> MatrixMultiply3/1
  Sum2/1 -> MatrixMultiply3/2
  (1-rho_s)*Sb/1(Out1) -> Sum2/1
  (2*rho_s*cos(theta)+2/3*rho_d)*Nb/1(Out1) -> Sum2/2
  MatrixMultiply3/1 -> F_sp/1
  Switch to compute only force of exposed surfaces/1(Out1) -> (2*rho_s*cos(theta)+2/3*rho_d)*Nb/1(In1), -PA*cos(theta)/1(In1)

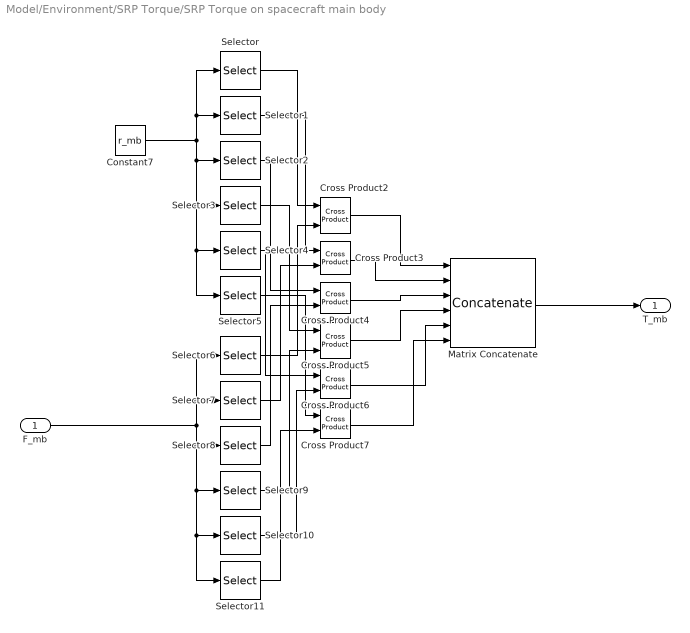
== system Model/Environment/SRP Torque/SRP Torque on spacecraft main body ==
  F_mb : Inport
  Constant7 : Constant  Value=r_mb
  Cross Product{2..7} (6 alike) : matrix_library/Cross Product
      settings: SourceProductBaseCode=SL
  Matrix Concatenate : Concatenate  NumInputs=6  Mode=Multidimensional array
  Selector : Selector  NumberOfDimensions=2  InputPortWidth=3  IndexOptions=Starting index (dialog),Starting index (dialog)  Indices=1,1  OutputSizes=1,3
  Selector1 : Selector  NumberOfDimensions=2  InputPortWidth=3  IndexOptions=Starting index (dialog),Starting index (dialog)  Indices=2,1  OutputSizes=1,3
  Selector10 : Selector  NumberOfDimensions=2  InputPortWidth=3  IndexOptions=Starting index (dialog),Starting index (dialog)  Indices=5,1  OutputSizes=1,3
  Selector11 : Selector  NumberOfDimensions=2  InputPortWidth=3  IndexOptions=Starting index (dialog),Starting index (dialog)  Indices=6,1  OutputSizes=1,3
  Selector2 : Selector  NumberOfDimensions=2  InputPortWidth=3  IndexOptions=Starting index (dialog),Starting index (dialog)  Indices=3,1  OutputSizes=1,3
  Selector3 : Selector  NumberOfDimensions=2  InputPortWidth=3  IndexOptions=Starting index (dialog),Starting index (dialog)  Indices=4,1  OutputSizes=1,3
  Selector4 : Selector  NumberOfDimensions=2  InputPortWidth=3  IndexOptions=Starting index (dialog),Starting index (dialog)  Indices=5,1  OutputSizes=1,3
  Selector5 : Selector  NumberOfDimensions=2  InputPortWidth=3  IndexOptions=Starting index (dialog),Starting index (dialog)  Indices=6,1  OutputSizes=1,3
  Selector6 : Selector  NumberOfDimensions=2  InputPortWidth=3  IndexOptions=Starting index (dialog),Starting index (dialog)  Indices=1,1  OutputSizes=1,3
  Selector7 : Selector  NumberOfDimensions=2  InputPortWidth=3  IndexOptions=Starting index (dialog),Starting index (dialog)  Indices=2,1  OutputSizes=1,3
  Selector8 : Selector  NumberOfDimensions=2  InputPortWidth=3  IndexOptions=Starting index (dialog),Starting index (dialog)  Indices=3,1  OutputSizes=1,3
  Selector9 : Selector  NumberOfDimensions=2  InputPortWidth=3  IndexOptions=Starting index (dialog),Starting index (dialog)  Indices=4,1  OutputSizes=1,3
  T_mb : Outport
  wires:
  Constant7/1 -> Selector2/1, Selector5/1, Selector4/1, Selector3/1, Selector1/1, Selector/1
  Selector5/1 -> Cross Product7/1
  Selector10/1 -> Cross Product6/2
  Selector/1 -> Cross Product2/1
  F_mb/1 -> Selector8/1, Selector11/1, Selector10/1, Selector9/1, Selector7/1, Selector6/1
  Matrix Concatenate/1 -> T_mb/1
  Selector7/1 -> Cross Product3/2
  Cross Product3/1 -> Matrix Concatenate/2
  Selector2/1 -> Cross Product4/1
  Selector9/1 -> Cross Product5/2
  Cross Product6/1 -> Matrix Concatenate/5
  Selector6/1 -> Cross Product2/2
  Selector1/1 -> Cross Product3/1
  Cross Product2/1 -> Matrix Concatenate/1
  Selector11/1 -> Cross Product7/2
  Cross Product5/1 -> Matrix Concatenate/4
  Selector4/1 -> Cross Product6/1
  Selector3/1 -> Cross Product5/1
  Cross Product4/1 -> Matrix Concatenate/3
  Cross Product7/1 -> Matrix Concatenate/6
  Selector8/1 -> Cross Product4/2

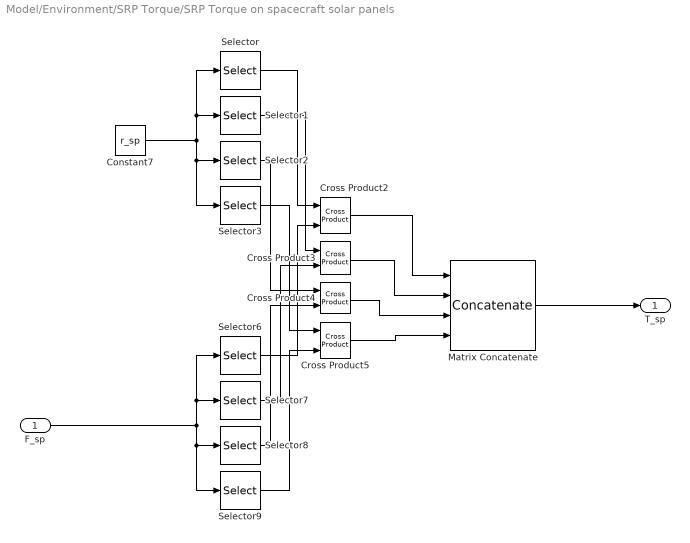
== system Model/Environment/SRP Torque/SRP Torque on spacecraft solar panels ==
  F_sp : Inport
  Constant7 : Constant  Value=r_sp
  Cross Product{2..5} (4 alike) : matrix_library/Cross Product
      settings: SourceProductBaseCode=SL
  Matrix Concatenate : Concatenate  NumInputs=4  Mode=Multidimensional array
  Selector : Selector  NumberOfDimensions=2  InputPortWidth=3  IndexOptions=Starting index (dialog),Starting index (dialog)  Indices=1,1  OutputSizes=1,3
  Selector1 : Selector  NumberOfDimensions=2  InputPortWidth=3  IndexOptions=Starting index (dialog),Starting index (dialog)  Indices=2,1  OutputSizes=1,3
  Selector2 : Selector  NumberOfDimensions=2  InputPortWidth=3  IndexOptions=Starting index (dialog),Starting index (dialog)  Indices=3,1  OutputSizes=1,3
  Selector3 : Selector  NumberOfDimensions=2  InputPortWidth=3  IndexOptions=Starting index (dialog),Starting index (dialog)  Indices=4,1  OutputSizes=1,3
  Selector6 : Selector  NumberOfDimensions=2  InputPortWidth=3  IndexOptions=Starting index (dialog),Starting index (dialog)  Indices=1,1  OutputSizes=1,3
  Selector7 : Selector  NumberOfDimensions=2  InputPortWidth=3  IndexOptions=Starting index (dialog),Starting index (dialog)  Indices=2,1  OutputSizes=1,3
  Selector8 : Selector  NumberOfDimensions=2  InputPortWidth=3  IndexOptions=Starting index (dialog),Starting index (dialog)  Indices=3,1  OutputSizes=1,3
  Selector9 : Selector  NumberOfDimensions=2  InputPortWidth=3  IndexOptions=Starting index (dialog),Starting index (dialog)  Indices=4,1  OutputSizes=1,3
  T_sp : Outport
  wires:
  Constant7/1 -> Selector2/1, Selector3/1, Selector1/1, Selector/1
  Selector/1 -> Cross Product2/1
  F_sp/1 -> Selector8/1, Selector9/1, Selector7/1, Selector6/1
  Matrix Concatenate/1 -> T_sp/1
  Selector7/1 -> Cross Product3/2
  Cross Product3/1 -> Matrix Concatenate/2
  Selector2/1 -> Cross Product4/1
  Selector9/1 -> Cross Product5/2
  Selector6/1 -> Cross Product2/2
  Selector1/1 -> Cross Product3/1
  Cross Product2/1 -> Matrix Concatenate/1
  Cross Product5/1 -> Matrix Concatenate/4
  Selector3/1 -> Cross Product5/1
  Cross Product4/1 -> Matrix Concatenate/3
  Selector8/1 -> Cross Product4/2

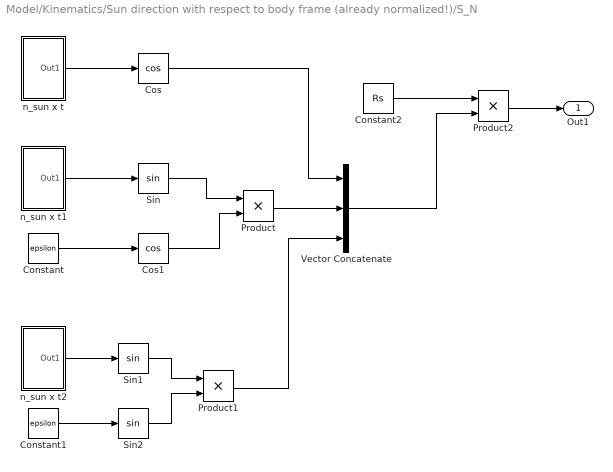
== system Model/Kinematics/Sun direction with respect to body frame (already normalized!)/S_N ==
  Constant : Constant  Value=epsilon
  Constant1 : Constant  Value=epsilon
  Constant2 : Constant  Value=Rs
  Cos : Trigonometry  Operator=cos
  Cos1 : Trigonometry  Operator=cos
  Product : Product
  Product1 : Product
  Product2 : Product
  Sin : Trigonometry
  Sin1 : Trigonometry
  Sin2 : Trigonometry
  Vector Concatenate : Concatenate  NumInputs=3
  n_sun x t : Subsystem
  n_sun x t1 : Subsystem
  n_sun x t2 : Subsystem
  Out1 : Outport
  wires:
  n_sun x t2/1(Out1) -> Sin1/1
  Vector Concatenate/1 -> Product2/2
  Sin2/1 -> Product1/2
  Sin/1 -> Product/1
  n_sun x t1/1(Out1) -> Sin/1
  Product1/1 -> Vector Concatenate/3
  Constant2/1 -> Product2/1
  Cos/1 -> Vector Concatenate/1
  Cos1/1 -> Product/2
  Product/1 -> Vector Concatenate/2
  n_sun x t/1(Out1) -> Cos/1
  Constant1/1 -> Sin2/1
  Sin1/1 -> Product1/1
  Constant/1 -> Cos1/1
  Product2/1 -> Out1/1

== system Model/Kinematics/radius of orbit in body frame and transformation matrix from inertial frame to body frame /finder of A_B//N(t) ==
  w : Inport
  Demux : Demux  Outputs=3
  Gain : Gain  Gain=-1
  Integrator1 : Integrator  InitialCondition=A0
  MatrixMultiply : Product  Multiplication=Matrix(*)
  w_hat : Subsystem
  A(t) : Outport
  wires:
  w/1 -> Demux/1
  Gain/1 -> MatrixMultiply/1
  Integrator1/1 -> A(t)/1, MatrixMultiply/2  "A(t)"
  w_hat/1(Out1) -> Gain/1
  Demux/3 -> w_hat/3(w_z)  "w_z"
  Demux/2 -> w_hat/2(w_y)  "w_y"
  Demux/1 -> w_hat/1(w_x)  "w_x"
  MatrixMultiply/1 -> Integrator1/1

== system Model/Kinematics/radius of orbit in body frame and transformation matrix from inertial frame to body frame /orthonormalization of matrix A(t) ==
  A(t) : Inport
  Gain7 : Gain  Gain=3/2
  Gain8 : Gain  Gain=1/2
  MatrixMultiply3 : Product  Multiplication=Matrix(*)
  MatrixMultiply4 : Product  Multiplication=Matrix(*)
  Sum : Sum  Inputs=+-
  Transpose : Math  Operator=transpose  SaturateOnIntegerOverflow=on
  A_orthonorm : Outport
  wires:
  Transpose/1 -> MatrixMultiply3/2
  MatrixMultiply4/1 -> Sum/2
  MatrixMultiply3/1 -> MatrixMultiply4/1
  Gain7/1 -> Sum/1
  Gain8/1 -> MatrixMultiply4/2  "A/2"
  A(t)/1 -> Gain8/1, Transpose/1, MatrixMultiply3/1, Gain7/1
  Sum/1 -> A_orthonorm/1  "A_orthonorm"

== system Model/Kinematics/radius of orbit in body frame and transformation matrix from inertial frame to body frame /radius of orbit in the inertial reference frame ==
  Product2 : Product
  Radius of orbit : Subsystem
  Theta : Subsystem
  vector [cos(theta); sin(theta)cos(i); sin(theta)sin(i)] : Subsystem
  theta : Outport
  r_N : Outport  Port=2
  R_orbit : Outport  Port=3
  wires:
  Theta/1(theta) -> vector [cos(theta); sin(theta)cos(i); sin(theta)sin(i)]/1(In1), theta/1, Radius of orbit/1(theta)
  Radius of orbit/1(R_orbit) -> Product2/1, R_orbit/1
  Product2/1 -> r_N/1
  vector [cos(theta); sin(theta)cos(i); sin(theta)sin(i)]/1(Out1) -> Product2/2

== system Model/Detumbling/Mangetic Torquer/w_hat/Subsystem ==
  w_x : Inport
  w_y : Inport  Port=2
  w_z : Inport  Port=3
  Constant2 : Constant  Value=v1
  Product2 : Product
  Vector Concatenate : Concatenate  NumInputs=3
  Out1 : Outport
  wires:
  Product2/1 -> Out1/1
  Vector Concatenate/1 -> Product2/1
  Constant2/1 -> Product2/2
  w_x/1 -> Vector Concatenate/1
  w_z/1 -> Vector Concatenate/2
  w_y/1 -> Vector Concatenate/3

== system Model/Detumbling/Mangetic Torquer/w_hat/Subsystem1 ==
  w_x : Inport
  w_y : Inport  Port=2
  w_z : Inport  Port=3
  Constant4 : Constant  Value=v2
  Product4 : Product
  Vector Concatenate2 : Concatenate  NumInputs=3
  Out1 : Outport
  wires:
  Constant4/1 -> Product4/2
  Vector Concatenate2/1 -> Product4/1
  Product4/1 -> Out1/1
  w_x/1 -> Vector Concatenate2/3
  w_y/1 -> Vector Concatenate2/2
  w_z/1 -> Vector Concatenate2/1

== system Model/Detumbling/Mangetic Torquer/w_hat/Subsystem2 ==
  w_x : Inport
  w_y : Inport  Port=2
  w_z : Inport  Port=3
  Constant3 : Constant  Value=v3
  Product3 : Product
  Vector Concatenate1 : Concatenate  NumInputs=3
  Out1 : Outport
  wires:
  Product3/1 -> Out1/1
  Constant3/1 -> Product3/2
  w_y/1 -> Vector Concatenate1/1
  Vector Concatenate1/1 -> Product3/1
  w_x/1 -> Vector Concatenate1/2
  w_z/1 -> Vector Concatenate1/3

== system Model/Environment/GG Torque/Gravity Gradient/creation of coefficient 3*mu_E//(R^3) ==
  In1 : Inport
  Constant : Constant  Value=3
  Constant1 : Constant  Value=mu_E
  Divide : Product  Inputs=*/
  Gain : Gain  Gain=3
  Power : Math  Operator=pow  SaturateOnIntegerOverflow=on
  Out1 : Outport
  wires:
  Divide/1 -> Out1/1
  Power/1 -> Divide/2
  Constant/1 -> Power/2
  In1/1 -> Power/1
  Constant1/1 -> Gain/1
  Gain/1 -> Divide/1

== system Model/Environment/GG Torque/Gravity Gradient/creation of vector c ==
  A_BL : Inport
  Constant : Constant  Value=unit  VectorParams1D=off
  MatrixMultiply3 : Product  Multiplication=Matrix(*)
  c : Outport
  wires:
  A_BL/1 -> MatrixMultiply3/1
  MatrixMultiply3/1 -> c/1
  Constant/1 -> MatrixMultiply3/2

== system Model/Environment/GG Torque/Transformation from A_B//N to A_B//L/creation of A L//N ==
  theta : Inport
  Matrix Concatenate : Concatenate  NumInputs=3  Mode=Multidimensional array  ConcatenateDimension=2
  first column of A_L/N : Subsystem
  second column of A_L/N : Subsystem
  third column of A_L/N : Subsystem
  A_L/N : Outport
  wires:
  second column of A_L/N/1(A_L/N (:,2)) -> Matrix Concatenate/2
  Matrix Concatenate/1 -> A_L/N/1
  first column of A_L/N/1(A_L/N (:,1)) -> Matrix Concatenate/1
  third column of A_L/N/1(A_L/N (:,3)) -> Matrix Concatenate/3
  theta/1 -> second column of A_L/N/1(theta), first column of A_L/N/1(theta)
